simulink model "Automated_model_features"  (R2020b)
settings: Solver=VariableStepAuto  StartTime=0.0  StopTime=10.0  RelTol=1e-3
undefined symbols (not defined in the file): sigbuilder_block
libraries: simulink x123
(part 2 of 2)

== system Automated_model_features/MODULES/Tire Pressure Monitoring System/TP_Monitoring/indicateHigh1 ==
  Enable : EnablePort
  Constant : Constant  Value=0
  Out1 : Outport
  wires:
  Constant/1 -> Out1/1

== system Automated_model_features/MODULES/Tire Pressure Monitoring System/TP_Monitoring/indicateHigh2 ==
  Enable : EnablePort
  Constant : Constant  Value=0
  Out1 : Outport
  wires:
  Constant/1 -> Out1/1

== system Automated_model_features/MODULES/Tire Pressure Monitoring System/TP_Monitoring/indicateHigh3 ==
  Enable : EnablePort
  Constant : Constant  Value=0
  Out1 : Outport
  wires:
  Constant/1 -> Out1/1

== system Automated_model_features/MODULES/Tire Pressure Monitoring System/TP_Monitoring/indicateHigh4 ==
  Enable : EnablePort
  Constant : Constant  Value=0
  Out1 : Outport
  wires:
  Constant/1 -> Out1/1

== system Automated_model_features/MODULES/Tire Pressure Monitoring System/TP_Monitoring/indicateLow1 ==
  Enable : EnablePort
  Constant : Constant
  Out1 : Outport
  wires:
  Constant/1 -> Out1/1

== system Automated_model_features/MODULES/Tire Pressure Monitoring System/TP_Monitoring/indicateLow2 ==
  Enable : EnablePort
  Constant : Constant
  Out1 : Outport
  wires:
  Constant/1 -> Out1/1

== system Automated_model_features/MODULES/Tire Pressure Monitoring System/TP_Monitoring/indicateLow3 ==
  Enable : EnablePort
  Constant : Constant
  Out1 : Outport
  wires:
  Constant/1 -> Out1/1

== system Automated_model_features/MODULES/Tire Pressure Monitoring System/TP_Monitoring/indicateLow4 ==
  Enable : EnablePort
  Constant : Constant
  Out1 : Outport
  wires:
  Constant/1 -> Out1/1

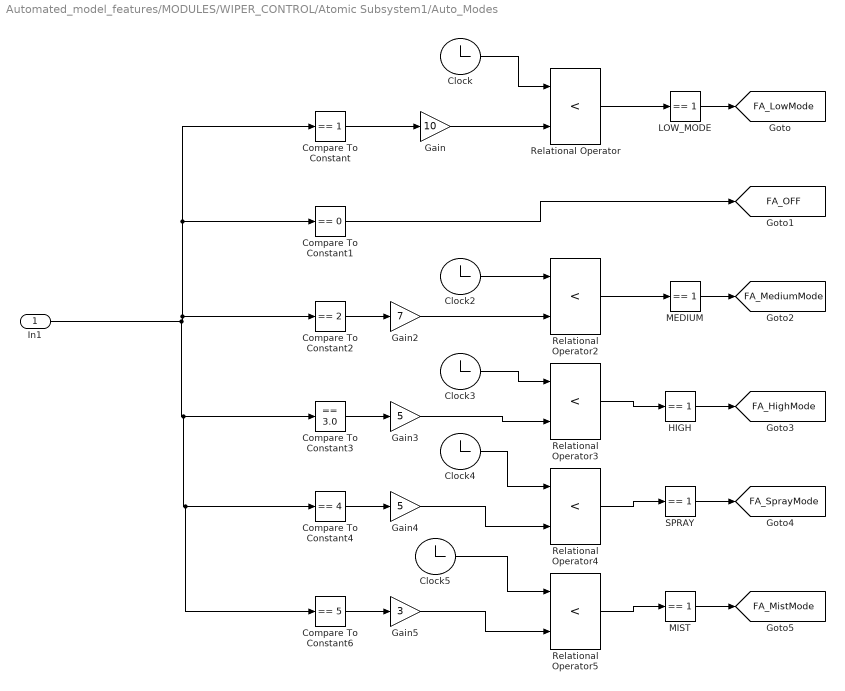
== system Automated_model_features/MODULES/WIPER_CONTROL/Atomic Subsystem1/Auto_Modes ==
  In1 : Inport
  Clock{,2..5} (5 alike) : Clock
      settings: Decimation=5
  Compare To Constant : simulink/Logic and Bit Operations/Compare To Constant  relop===  const=1  OutDataTypeStr=boolean
  Compare To Constant1 : simulink/Logic and Bit Operations/Compare To Constant  relop===  const=0  OutDataTypeStr=boolean
  Compare To Constant2 : simulink/Logic and Bit Operations/Compare To Constant  relop===  const=2  OutDataTypeStr=boolean
  Compare To Constant3 : simulink/Logic and Bit Operations/Compare To Constant  relop===  const=3.0  OutDataTypeStr=boolean
  Compare To Constant4 : simulink/Logic and Bit Operations/Compare To Constant  relop===  const=4  OutDataTypeStr=boolean
  Compare To Constant6 : simulink/Logic and Bit Operations/Compare To Constant  relop===  const=5  OutDataTypeStr=boolean
  Gain : Gain  Gain=10
  Gain2 : Gain  Gain=7
  Gain3 : Gain  Gain=5
  Gain4 : Gain  Gain=5
  Gain5 : Gain  Gain=3
  HIGH : simulink/Logic and Bit Operations/Compare To Constant  relop===  const=1  OutDataTypeStr=boolean
  LOW_MODE : simulink/Logic and Bit Operations/Compare To Constant  relop===  const=1  OutDataTypeStr=boolean
  MEDIUM : simulink/Logic and Bit Operations/Compare To Constant  relop===  const=1  OutDataTypeStr=boolean
  MIST : simulink/Logic and Bit Operations/Compare To Constant  relop===  const=1  OutDataTypeStr=boolean
  Relational Operator{,2..5} (5 alike) : RelationalOperator  Operator=<  OutDataTypeStr=boolean  RndMeth=Simplest
  SPRAY : simulink/Logic and Bit Operations/Compare To Constant  relop===  const=1  OutDataTypeStr=boolean
  tag scope: FA_HighMode=global, FA_LowMode=global, FA_MediumMode=global, FA_MistMode=global, FA_OFF=global, FA_SprayMode=global
  wires:
  In1/1 -> Compare To Constant6/1, Compare To Constant4/1, Compare To Constant3/1, Compare To Constant2/1, Compare To Constant/1, Compare To Constant1/1
  Clock/1 -> Relational Operator/1
  Relational Operator/1 -> LOW_MODE/1
  Gain/1 -> Relational Operator/2
  Compare To Constant/1 -> Gain/1
  Clock2/1 -> Relational Operator2/1
  Gain2/1 -> Relational Operator2/2
  Compare To Constant2/1 -> Gain2/1
  Clock3/1 -> Relational Operator3/1
  Gain3/1 -> Relational Operator3/2
  Compare To Constant3/1 -> Gain3/1
  Gain4/1 -> Relational Operator4/2
  Clock4/1 -> Relational Operator4/1
  Compare To Constant4/1 -> Gain4/1
  LOW_MODE/1 -> [FA_LowMode]
  MEDIUM/1 -> [FA_MediumMode]
  Relational Operator2/1 -> MEDIUM/1
  HIGH/1 -> [FA_HighMode]
  Relational Operator3/1 -> HIGH/1
  SPRAY/1 -> [FA_SprayMode]
  Relational Operator4/1 -> SPRAY/1
  Compare To Constant1/1 -> [FA_OFF]
  Relational Operator5/1 -> MIST/1
  Gain5/1 -> Relational Operator5/2
  Clock5/1 -> Relational Operator5/1
  MIST/1 -> [FA_MistMode]
  Compare To Constant6/1 -> Gain5/1

== system Automated_model_features/MODULES/WIPER_CONTROL/Atomic Subsystem1/Manual_mode ==
  In1 : Inport
  Bw30_60 : Logic  IconShape=distinctive  AllPortsSameDT=off  OutDataTypeStr=boolean
  Bw60_100 : Logic  IconShape=distinctive  AllPortsSameDT=off  OutDataTypeStr=boolean
  Compare To Constant1 : simulink/Logic and Bit Operations/Compare To Constant  relop=>  const=30  OutDataTypeStr=boolean
  Compare To Constant2 : simulink/Logic and Bit Operations/Compare To Constant  relop=<=  const=60  OutDataTypeStr=boolean
  Compare To Constant3 : simulink/Logic and Bit Operations/Compare To Constant  relop=>  const=60  OutDataTypeStr=boolean
  Compare To Constant4 : simulink/Logic and Bit Operations/Compare To Constant  relop=<=  const=100  OutDataTypeStr=boolean
  Display : Display
  LessThan30 : simulink/Logic and Bit Operations/Compare To Constant  relop=<=  const=30  OutDataTypeStr=boolean
  Slider : SliderBlock
  String Constant : StringConstant  String="\"Undefined!\""
  Switch : Switch  Criteria=u2 > Threshold  Threshold=5
  tag scope: FM_Bw30_60=global, FM_Bw60_100=global, FM_lessthan30=global
  wires:
  Compare To Constant1/1 -> Bw30_60/1
  Bw30_60/1 -> [FM_Bw30_60]
  [FC_ManualInput] -> Compare To Constant4/1, Compare To Constant3/1, Compare To Constant2/1, Compare To Constant1/1, LessThan30/1, Switch/1
  Compare To Constant4/1 -> Bw60_100/2
  LessThan30/1 -> [FM_lessthan30]
  Switch/1 -> Display/1
  Compare To Constant3/1 -> Bw60_100/1
  Bw60_100/1 -> [FM_Bw60_100]
  Compare To Constant2/1 -> Bw30_60/2
  In1/1 -> Switch/2
  String Constant/1 -> Switch/3

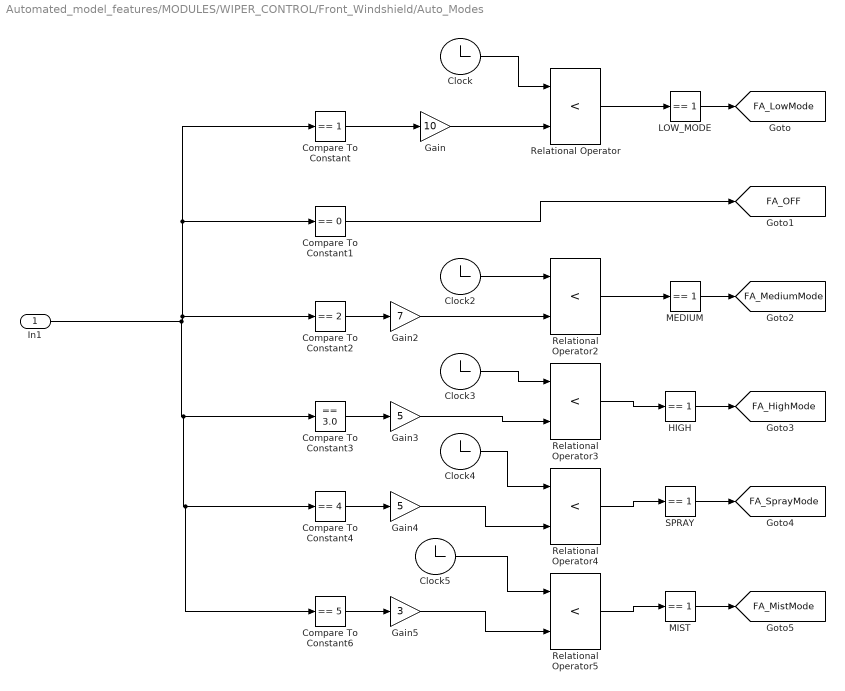
== system Automated_model_features/MODULES/WIPER_CONTROL/Front_Windshield/Auto_Modes ==
  In1 : Inport
  Clock{,2..5} (5 alike) : Clock
      settings: Decimation=5
  Compare To Constant : simulink/Logic and Bit Operations/Compare To Constant  relop===  const=1  OutDataTypeStr=boolean
  Compare To Constant1 : simulink/Logic and Bit Operations/Compare To Constant  relop===  const=0  OutDataTypeStr=boolean
  Compare To Constant2 : simulink/Logic and Bit Operations/Compare To Constant  relop===  const=2  OutDataTypeStr=boolean
  Compare To Constant3 : simulink/Logic and Bit Operations/Compare To Constant  relop===  const=3.0  OutDataTypeStr=boolean
  Compare To Constant4 : simulink/Logic and Bit Operations/Compare To Constant  relop===  const=4  OutDataTypeStr=boolean
  Compare To Constant6 : simulink/Logic and Bit Operations/Compare To Constant  relop===  const=5  OutDataTypeStr=boolean
  Gain : Gain  Gain=10
  Gain2 : Gain  Gain=7
  Gain3 : Gain  Gain=5
  Gain4 : Gain  Gain=5
  Gain5 : Gain  Gain=3
  HIGH : simulink/Logic and Bit Operations/Compare To Constant  relop===  const=1  OutDataTypeStr=boolean
  LOW_MODE : simulink/Logic and Bit Operations/Compare To Constant  relop===  const=1  OutDataTypeStr=boolean
  MEDIUM : simulink/Logic and Bit Operations/Compare To Constant  relop===  const=1  OutDataTypeStr=boolean
  MIST : simulink/Logic and Bit Operations/Compare To Constant  relop===  const=1  OutDataTypeStr=boolean
  Relational Operator{,2..5} (5 alike) : RelationalOperator  Operator=<  OutDataTypeStr=boolean  RndMeth=Simplest
  SPRAY : simulink/Logic and Bit Operations/Compare To Constant  relop===  const=1  OutDataTypeStr=boolean
  tag scope: FA_HighMode=global, FA_LowMode=global, FA_MediumMode=global, FA_MistMode=global, FA_OFF=global, FA_SprayMode=global
  wires:
  In1/1 -> Compare To Constant6/1, Compare To Constant4/1, Compare To Constant3/1, Compare To Constant2/1, Compare To Constant/1, Compare To Constant1/1
  Clock/1 -> Relational Operator/1
  Relational Operator/1 -> LOW_MODE/1
  Gain/1 -> Relational Operator/2
  Compare To Constant/1 -> Gain/1
  Clock2/1 -> Relational Operator2/1
  Gain2/1 -> Relational Operator2/2
  Compare To Constant2/1 -> Gain2/1
  Clock3/1 -> Relational Operator3/1
  Gain3/1 -> Relational Operator3/2
  Compare To Constant3/1 -> Gain3/1
  Gain4/1 -> Relational Operator4/2
  Clock4/1 -> Relational Operator4/1
  Compare To Constant4/1 -> Gain4/1
  LOW_MODE/1 -> [FA_LowMode]
  MEDIUM/1 -> [FA_MediumMode]
  Relational Operator2/1 -> MEDIUM/1
  HIGH/1 -> [FA_HighMode]
  Relational Operator3/1 -> HIGH/1
  SPRAY/1 -> [FA_SprayMode]
  Relational Operator4/1 -> SPRAY/1
  Compare To Constant1/1 -> [FA_OFF]
  Relational Operator5/1 -> MIST/1
  Gain5/1 -> Relational Operator5/2
  Clock5/1 -> Relational Operator5/1
  MIST/1 -> [FA_MistMode]
  Compare To Constant6/1 -> Gain5/1

== system Automated_model_features/MODULES/WIPER_CONTROL/Front_Windshield/Manual_mode ==
  In1 : Inport
  Bw30_60 : Logic  IconShape=distinctive  AllPortsSameDT=off  OutDataTypeStr=boolean
  Bw60_100 : Logic  IconShape=distinctive  AllPortsSameDT=off  OutDataTypeStr=boolean
  Compare To Constant1 : simulink/Logic and Bit Operations/Compare To Constant  relop=>  const=30  OutDataTypeStr=boolean
  Compare To Constant2 : simulink/Logic and Bit Operations/Compare To Constant  relop=<=  const=60  OutDataTypeStr=boolean
  Compare To Constant3 : simulink/Logic and Bit Operations/Compare To Constant  relop=>  const=60  OutDataTypeStr=boolean
  Compare To Constant4 : simulink/Logic and Bit Operations/Compare To Constant  relop=<=  const=100  OutDataTypeStr=boolean
  Display : Display
  LessThan30 : simulink/Logic and Bit Operations/Compare To Constant  relop=<=  const=30  OutDataTypeStr=boolean
  Slider : SliderBlock
  String Constant : StringConstant  String="\"Undefined!\""
  Switch : Switch  Criteria=u2 > Threshold  Threshold=5
  tag scope: FM_Bw30_60=global, FM_Bw60_100=global, FM_lessthan30=global
  wires:
  Compare To Constant1/1 -> Bw30_60/1
  Bw30_60/1 -> [FM_Bw30_60]
  [FC_ManualInput] -> Compare To Constant4/1, Compare To Constant3/1, Compare To Constant2/1, Compare To Constant1/1, LessThan30/1, Switch/1
  Compare To Constant4/1 -> Bw60_100/2
  LessThan30/1 -> [FM_lessthan30]
  Switch/1 -> Display/1
  Compare To Constant3/1 -> Bw60_100/1
  Bw60_100/1 -> [FM_Bw60_100]
  Compare To Constant2/1 -> Bw30_60/2
  In1/1 -> Switch/2
  String Constant/1 -> Switch/3

== system Automated_model_features/MODULES/WIPER_CONTROL/Wiper_Control/Atomic Subsystem ==
  Inport : Inport
  Clock : Clock
      settings: Decimation=5
  Compare To Constant : simulink/Logic and Bit Operations/Compare To Constant  relop===  const=1  OutDataTypeStr=boolean
  Compare To Constant5 : simulink/Logic and Bit Operations/Compare To Constant  relop===  const=1  OutDataTypeStr=boolean
  Gain : Gain  Gain=10
  Relational Operator : RelationalOperator  Operator=<  OutDataTypeStr=boolean  RndMeth=Simplest
  tag scope: BW_Display=global
  wires:
  Compare To Constant5/1 -> [BW_Display]
  Inport/1 -> Compare To Constant/1
  Gain/1 -> Relational Operator/2
  Clock/1 -> Relational Operator/1
  Relational Operator/1 -> Compare To Constant5/1
  Compare To Constant/1 -> Gain/1

== system Automated_model_features/MODULES/WIPER_CONTROL/Wiper_Control/Atomic Subsystem1 ==
  Inport : Inport
  Auto_Modes : Subsystem
  Display : Display
  Manual_mode : Subsystem
  wires:
  [FW_Modes] -> Manual_mode/1(In1), Auto_Modes/1(In1)
  Inport/1 -> Display/1

== system Automated_model_features/MODULES/WIPER_CONTROL/Wiper_Control/Back_Windshield ==
  Lamp : LampBlock

== system Automated_model_features/MODULES/WIPER_CONTROL/Wiper_Control/Front_Windshield ==
  Enable : EnablePort
  Auto_Modes : Subsystem
  Manual_mode : Subsystem
  Rotary Switch : RotarySwitchBlock  Commented=on
      settings: Values={{'Off', 'Low', 'Medium', 'High', 'Spray', 'Manual', 'MistMode'}, [0 1 2 3 4 5 6]}
  wires:
  [FW_Modes] -> Manual_mode/1(In1), Auto_Modes/1(In1)

== system Automated_model_features/MODULES/sunroof/Subsystem/Enabled Subsystem ==
  In1 : Inport
  Enable : EnablePort
  Outport : Outport
  wires:
  In1/1 -> Outport/1

== system Automated_model_features/MODULES/sunroof/Subsystem1/Enabled Subsystem1 ==
  In1 : Inport
  Enable : EnablePort
  Outport : Outport
  wires:
  In1/1 -> Outport/1

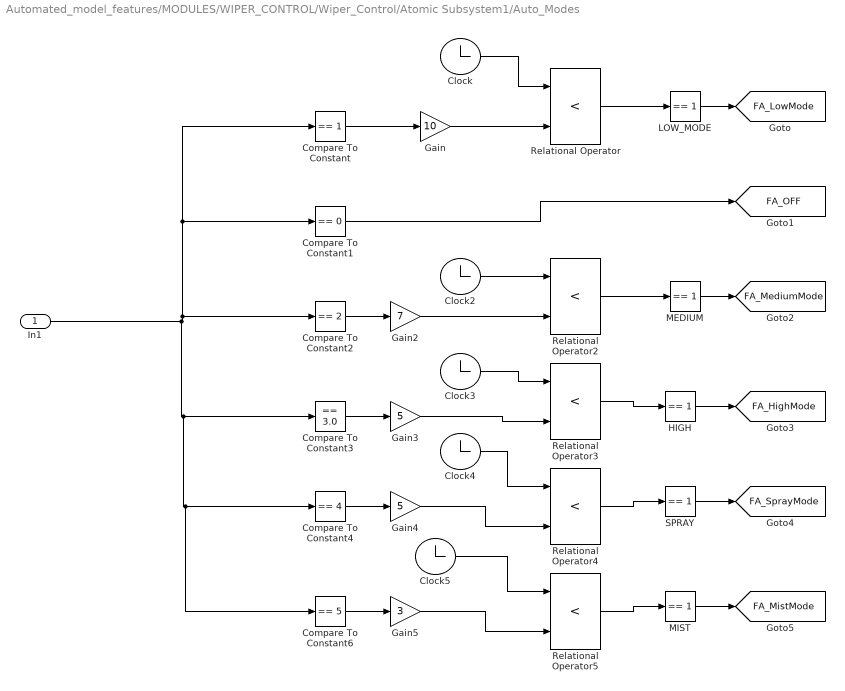
== system Automated_model_features/MODULES/WIPER_CONTROL/Wiper_Control/Atomic Subsystem1/Auto_Modes ==
  In1 : Inport
  Clock{,2..5} (5 alike) : Clock
      settings: Decimation=5
  Compare To Constant : simulink/Logic and Bit Operations/Compare To Constant  relop===  const=1  OutDataTypeStr=boolean
  Compare To Constant1 : simulink/Logic and Bit Operations/Compare To Constant  relop===  const=0  OutDataTypeStr=boolean
  Compare To Constant2 : simulink/Logic and Bit Operations/Compare To Constant  relop===  const=2  OutDataTypeStr=boolean
  Compare To Constant3 : simulink/Logic and Bit Operations/Compare To Constant  relop===  const=3.0  OutDataTypeStr=boolean
  Compare To Constant4 : simulink/Logic and Bit Operations/Compare To Constant  relop===  const=4  OutDataTypeStr=boolean
  Compare To Constant6 : simulink/Logic and Bit Operations/Compare To Constant  relop===  const=5  OutDataTypeStr=boolean
  Gain : Gain  Gain=10
  Gain2 : Gain  Gain=7
  Gain3 : Gain  Gain=5
  Gain4 : Gain  Gain=5
  Gain5 : Gain  Gain=3
  HIGH : simulink/Logic and Bit Operations/Compare To Constant  relop===  const=1  OutDataTypeStr=boolean
  LOW_MODE : simulink/Logic and Bit Operations/Compare To Constant  relop===  const=1  OutDataTypeStr=boolean
  MEDIUM : simulink/Logic and Bit Operations/Compare To Constant  relop===  const=1  OutDataTypeStr=boolean
  MIST : simulink/Logic and Bit Operations/Compare To Constant  relop===  const=1  OutDataTypeStr=boolean
  Relational Operator{,2..5} (5 alike) : RelationalOperator  Operator=<  OutDataTypeStr=boolean  RndMeth=Simplest
  SPRAY : simulink/Logic and Bit Operations/Compare To Constant  relop===  const=1  OutDataTypeStr=boolean
  tag scope: FA_HighMode=global, FA_LowMode=global, FA_MediumMode=global, FA_MistMode=global, FA_OFF=global, FA_SprayMode=global
  wires:
  In1/1 -> Compare To Constant6/1, Compare To Constant4/1, Compare To Constant3/1, Compare To Constant2/1, Compare To Constant/1, Compare To Constant1/1
  Clock/1 -> Relational Operator/1
  Relational Operator/1 -> LOW_MODE/1
  Gain/1 -> Relational Operator/2
  Compare To Constant/1 -> Gain/1
  Clock2/1 -> Relational Operator2/1
  Gain2/1 -> Relational Operator2/2
  Compare To Constant2/1 -> Gain2/1
  Clock3/1 -> Relational Operator3/1
  Gain3/1 -> Relational Operator3/2
  Compare To Constant3/1 -> Gain3/1
  Gain4/1 -> Relational Operator4/2
  Clock4/1 -> Relational Operator4/1
  Compare To Constant4/1 -> Gain4/1
  LOW_MODE/1 -> [FA_LowMode]
  MEDIUM/1 -> [FA_MediumMode]
  Relational Operator2/1 -> MEDIUM/1
  HIGH/1 -> [FA_HighMode]
  Relational Operator3/1 -> HIGH/1
  SPRAY/1 -> [FA_SprayMode]
  Relational Operator4/1 -> SPRAY/1
  Compare To Constant1/1 -> [FA_OFF]
  Relational Operator5/1 -> MIST/1
  Gain5/1 -> Relational Operator5/2
  Clock5/1 -> Relational Operator5/1
  MIST/1 -> [FA_MistMode]
  Compare To Constant6/1 -> Gain5/1

== system Automated_model_features/MODULES/WIPER_CONTROL/Wiper_Control/Atomic Subsystem1/Manual_mode ==
  In1 : Inport
  Bw30_60 : Logic  IconShape=distinctive  AllPortsSameDT=off  OutDataTypeStr=boolean
  Bw60_100 : Logic  IconShape=distinctive  AllPortsSameDT=off  OutDataTypeStr=boolean
  Compare To Constant1 : simulink/Logic and Bit Operations/Compare To Constant  relop=>  const=30  OutDataTypeStr=boolean
  Compare To Constant2 : simulink/Logic and Bit Operations/Compare To Constant  relop=<=  const=60  OutDataTypeStr=boolean
  Compare To Constant3 : simulink/Logic and Bit Operations/Compare To Constant  relop=>  const=60  OutDataTypeStr=boolean
  Compare To Constant4 : simulink/Logic and Bit Operations/Compare To Constant  relop=<=  const=100  OutDataTypeStr=boolean
  Display : Display
  LessThan30 : simulink/Logic and Bit Operations/Compare To Constant  relop=<=  const=30  OutDataTypeStr=boolean
  Slider : SliderBlock
  String Constant : StringConstant  String="\"Undefined!\""
  Switch : Switch  Criteria=u2 > Threshold  Threshold=5
  tag scope: FM_Bw30_60=global, FM_Bw60_100=global, FM_lessthan30=global
  wires:
  Compare To Constant1/1 -> Bw30_60/1
  Bw30_60/1 -> [FM_Bw30_60]
  [FC_ManualInput] -> Compare To Constant4/1, Compare To Constant3/1, Compare To Constant2/1, Compare To Constant1/1, LessThan30/1, Switch/1
  Compare To Constant4/1 -> Bw60_100/2
  LessThan30/1 -> [FM_lessthan30]
  Switch/1 -> Display/1
  Compare To Constant3/1 -> Bw60_100/1
  Bw60_100/1 -> [FM_Bw60_100]
  Compare To Constant2/1 -> Bw30_60/2
  In1/1 -> Switch/2
  String Constant/1 -> Switch/3

== system Automated_model_features/MODULES/WIPER_CONTROL/Wiper_Control/Front_Windshield/Auto_Modes ==
  In1 : Inport
  Clock{,2..5} (5 alike) : Clock
      settings: Decimation=5
  Compare To Constant : simulink/Logic and Bit Operations/Compare To Constant  relop===  const=1  OutDataTypeStr=boolean
  Compare To Constant1 : simulink/Logic and Bit Operations/Compare To Constant  relop===  const=0  OutDataTypeStr=boolean
  Compare To Constant2 : simulink/Logic and Bit Operations/Compare To Constant  relop===  const=2  OutDataTypeStr=boolean
  Compare To Constant3 : simulink/Logic and Bit Operations/Compare To Constant  relop===  const=3.0  OutDataTypeStr=boolean
  Compare To Constant4 : simulink/Logic and Bit Operations/Compare To Constant  relop===  const=4  OutDataTypeStr=boolean
  Compare To Constant6 : simulink/Logic and Bit Operations/Compare To Constant  relop===  const=5  OutDataTypeStr=boolean
  Gain : Gain  Gain=10
  Gain2 : Gain  Gain=7
  Gain3 : Gain  Gain=5
  Gain4 : Gain  Gain=5
  Gain5 : Gain  Gain=3
  HIGH : simulink/Logic and Bit Operations/Compare To Constant  relop===  const=1  OutDataTypeStr=boolean
  LOW_MODE : simulink/Logic and Bit Operations/Compare To Constant  relop===  const=1  OutDataTypeStr=boolean
  MEDIUM : simulink/Logic and Bit Operations/Compare To Constant  relop===  const=1  OutDataTypeStr=boolean
  MIST : simulink/Logic and Bit Operations/Compare To Constant  relop===  const=1  OutDataTypeStr=boolean
  Relational Operator{,2..5} (5 alike) : RelationalOperator  Operator=<  OutDataTypeStr=boolean  RndMeth=Simplest
  SPRAY : simulink/Logic and Bit Operations/Compare To Constant  relop===  const=1  OutDataTypeStr=boolean
  tag scope: FA_HighMode=global, FA_LowMode=global, FA_MediumMode=global, FA_MistMode=global, FA_OFF=global, FA_SprayMode=global
  wires:
  In1/1 -> Compare To Constant6/1, Compare To Constant4/1, Compare To Constant3/1, Compare To Constant2/1, Compare To Constant/1, Compare To Constant1/1
  Clock/1 -> Relational Operator/1
  Relational Operator/1 -> LOW_MODE/1
  Gain/1 -> Relational Operator/2
  Compare To Constant/1 -> Gain/1
  Clock2/1 -> Relational Operator2/1
  Gain2/1 -> Relational Operator2/2
  Compare To Constant2/1 -> Gain2/1
  Clock3/1 -> Relational Operator3/1
  Gain3/1 -> Relational Operator3/2
  Compare To Constant3/1 -> Gain3/1
  Gain4/1 -> Relational Operator4/2
  Clock4/1 -> Relational Operator4/1
  Compare To Constant4/1 -> Gain4/1
  LOW_MODE/1 -> [FA_LowMode]
  MEDIUM/1 -> [FA_MediumMode]
  Relational Operator2/1 -> MEDIUM/1
  HIGH/1 -> [FA_HighMode]
  Relational Operator3/1 -> HIGH/1
  SPRAY/1 -> [FA_SprayMode]
  Relational Operator4/1 -> SPRAY/1
  Compare To Constant1/1 -> [FA_OFF]
  Relational Operator5/1 -> MIST/1
  Gain5/1 -> Relational Operator5/2
  Clock5/1 -> Relational Operator5/1
  MIST/1 -> [FA_MistMode]
  Compare To Constant6/1 -> Gain5/1

== system Automated_model_features/MODULES/WIPER_CONTROL/Wiper_Control/Front_Windshield/Manual_mode ==
  In1 : Inport
  Bw30_60 : Logic  IconShape=distinctive  AllPortsSameDT=off  OutDataTypeStr=boolean
  Bw60_100 : Logic  IconShape=distinctive  AllPortsSameDT=off  OutDataTypeStr=boolean
  Compare To Constant1 : simulink/Logic and Bit Operations/Compare To Constant  relop=>  const=30  OutDataTypeStr=boolean
  Compare To Constant2 : simulink/Logic and Bit Operations/Compare To Constant  relop=<=  const=60  OutDataTypeStr=boolean
  Compare To Constant3 : simulink/Logic and Bit Operations/Compare To Constant  relop=>  const=60  OutDataTypeStr=boolean
  Compare To Constant4 : simulink/Logic and Bit Operations/Compare To Constant  relop=<=  const=100  OutDataTypeStr=boolean
  Display : Display
  LessThan30 : simulink/Logic and Bit Operations/Compare To Constant  relop=<=  const=30  OutDataTypeStr=boolean
  Slider : SliderBlock
  String Constant : StringConstant  String="\"Undefined!\""
  Switch : Switch  Criteria=u2 > Threshold  Threshold=5
  tag scope: FM_Bw30_60=global, FM_Bw60_100=global, FM_lessthan30=global
  wires:
  Compare To Constant1/1 -> Bw30_60/1
  Bw30_60/1 -> [FM_Bw30_60]
  [FC_ManualInput] -> Compare To Constant4/1, Compare To Constant3/1, Compare To Constant2/1, Compare To Constant1/1, LessThan30/1, Switch/1
  Compare To Constant4/1 -> Bw60_100/2
  LessThan30/1 -> [FM_lessthan30]
  Switch/1 -> Display/1
  Compare To Constant3/1 -> Bw60_100/1
  Bw60_100/1 -> [FM_Bw60_100]
  Compare To Constant2/1 -> Bw30_60/2
  In1/1 -> Switch/2
  String Constant/1 -> Switch/3

== stateflow chart Automated_model_features/MODULES/ALARM_SYSTEM/Pre_Alarm ==
  state RKE1
    entry:
  state DELAY_3
    entry:
    data1 = 1;
  state DELAY_2
    entry:
    counter=0;
    counter = counter +1;
    data1 = 0;
  (default) -> RKE1
  RKE1 -> DELAY_3 [order 2] : [data==1]
  RKE1 -> DELAY_2 [order 1] : [data==0]
  DELAY_2 -> DELAY_2 : [counter~=10]
  data: data input; data1 output; counter local

== stateflow chart Automated_model_features/MODULES/sunroof/enabling system/Chart ==
  state stage1
    entry:
    enableO=0;
    enableC=0;
  state stage3
    entry:
    enableO=1;
    enableC=0;
  state stage2
    entry:
    enableO=0;
    enableC=1;
  (default) -> stage1
  stage1 -> stage3 [order 3] : [openButton ==1 && closeButton==0]
  stage1 -> stage2 [order 1] : [openButton ==0 && closeButton==1]
  stage2 -> stage1 : [(openButton ==1 && closeButton==1) || (openButton ==0 && closeButton==0)]
  stage3 -> stage1 : [(openButton ==1 && closeButton==1) || (openButton ==0 && closeButton==0)]
  stage1 -> stage1 [order 2] : [(openButton ==1 && closeButton==1) || (openButton ==0 && closeButton==0)]
  data: closeButton input; openButton input; enableC output; enableO output

== matlab function Automated_model_features/MODULES/AIRBAGSYSTEM/ActivateAirBagSensor ==
  data: SuddenDeceleration input; AirBagSensor output
function AirBagSensor  = fcn(SuddenDeceleration)
if SuddenDeceleration == 1
         %Front airbag active
   AirBagSensor = 1;
else 
   AirBagSensor = 0;   
end

== matlab function Automated_model_features/MODULES/AIRBAGSYSTEM/FrontAirBagActivation/WeightSensor ==
  data: driver input; DRIVER output; l_front input; L_FRONT output; l_rear input; r_rear input; L_REAR output; R_REAR output
function [DRIVER,L_FRONT,L_REAR,R_REAR] = fcn(driver, l_front,l_rear,r_rear)
    if (driver==0 && l_front==0 && l_rear==0 && r_rear==1)      %0001
        DRIVER=0;
        L_FRONT=0;
        L_REAR=0;
        R_REAR=1;
    
    elseif (driver==0 && l_front==0 && l_rear==1 && r_rear==0)
        DRIVER=0;
        L_FRONT=0;
        L_REAR=1;
        R_REAR=0;
    
    elseif (driver==0 && l_front==0 && l_rear==1 && r_rear==1)
        DRIVER=0;
        L_FRONT=0;
        L_REAR=1;
        R_REAR=1;

    elseif (driver==0 && l_front==1 && l_rear==0 && r_rear==0)
        DRIVER=0;
        L_FRONT=1;
        L_REAR=0;
        R_REAR=0;
    
    elseif (driver==0 && l_front==1 && l_rear==0 && r_rear==1)
        DRIVER=0;
        L_FRONT=1;
        L_REAR=0;
        R_REAR=1;
    
    elseif (driver==0 && l_front==1 && l_rear==1 && r_rear==0)
        DRIVER=0;
        L_FRONT=1;
        L_REAR=1;
        R_REAR=0;
    
    elseif (driver==0 && l_front==1 && l_rear==1 && r_rear==1)
        DRIVER=0;
        L_FRONT=1;
        L_REAR=1;
        R_REAR=1;
    
    elseif (driver==1 && l_front==0 && l_rear==0 && r_rear==0)
        DRIVER=1;
        L_FRONT=0;
        L_REAR=0;
        R_REAR=0;
    
    elseif (driver==1 && l_front==0 && l_rear==0 && r_rear==1)
        DRIVER=1;
        L_FRONT=0;
        L_REAR=0;
        R_REAR=1;
    
    elseif (driver==1 && l_front==0 && l_rear==1 && r_rear==0)
        DRIVER=1;
        L_FRONT=0;
        L_REAR=1;
        R_REAR=0;
    
    elseif (driver==1 && l_front==0 && l_rear==1 && r_rear==1)
        DRIVER=1;
        L_FRONT=0;
        L_REAR=1;
        R_REAR=1;
    
    elseif (driver==1 && l_front==1 && l_rear==0 && r_rear==0)
        DRIVER=1;
        L_FRONT=1;
        L_REAR=0;
        R_REAR=0;
    
    elseif (driver==1 && l_front==1 && l_rear==0 && r_rear==1)
        DRIVER=1;
        L_FRONT=1;
        L_REAR=0;
        R_REAR=1;
    
    elseif (driver==1 && l_front==1 && l_rear==1 && r_rear==0)
        DRIVER=1;
        L_FRONT=1;
        L_REAR=1;
        R_REAR=0;
    
    elseif (driver==1 && l_front==1 && l_rear==1 && r_rear==1)
        DRIVER=1;
        L_FRONT=1;
        L_REAR=1;
        R_REAR=1;
    
    else
        DRIVER=0;
        L_FRONT=0;
        L_REAR=0;
        R_REAR=0;
    end

== matlab function Automated_model_features/MODULES/AIRBAGSYSTEM/SideAirBagActivation1/WeightSensor ==
  data: driver input; DRIVER output; l_front input; L_FRONT output; l_rear input; r_rear input; L_REAR output; R_REAR output
function [DRIVER,L_FRONT,L_REAR,R_REAR] = fcn(driver, l_front,l_rear,r_rear)
    if (driver==0 && l_front==0 && l_rear==0 && r_rear==1)      %0001
        DRIVER=0;
        L_FRONT=0;
        L_REAR=0;
        R_REAR=1;
    
    elseif (driver==0 && l_front==0 && l_rear==1 && r_rear==0)
        DRIVER=0;
        L_FRONT=0;
        L_REAR=1;
        R_REAR=0;
    
    elseif (driver==0 && l_front==0 && l_rear==1 && r_rear==1)
        DRIVER=0;
        L_FRONT=0;
        L_REAR=1;
        R_REAR=1;

    elseif (driver==0 && l_front==1 && l_rear==0 && r_rear==0)
        DRIVER=0;
        L_FRONT=1;
        L_REAR=0;
        R_REAR=0;
    
    elseif (driver==0 && l_front==1 && l_rear==0 && r_rear==1)
        DRIVER=0;
        L_FRONT=1;
        L_REAR=0;
        R_REAR=1;
    
    elseif (driver==0 && l_front==1 && l_rear==1 && r_rear==0)
        DRIVER=0;
        L_FRONT=1;
        L_REAR=1;
        R_REAR=0;
    
    elseif (driver==0 && l_front==1 && l_rear==1 && r_rear==1)
        DRIVER=0;
        L_FRONT=1;
        L_REAR=1;
        R_REAR=1;
    
    elseif (driver==1 && l_front==0 && l_rear==0 && r_rear==0)
        DRIVER=1;
        L_FRONT=0;
        L_REAR=0;
        R_REAR=0;
    
    elseif (driver==1 && l_front==0 && l_rear==0 && r_rear==1)
        DRIVER=1;
        L_FRONT=0;
        L_REAR=0;
        R_REAR=1;
    
    elseif (driver==1 && l_front==0 && l_rear==1 && r_rear==0)
        DRIVER=1;
        L_FRONT=0;
        L_REAR=1;
        R_REAR=0;
    
    elseif (driver==1 && l_front==0 && l_rear==1 && r_rear==1)
        DRIVER=1;
        L_FRONT=0;
        L_REAR=1;
        R_REAR=1;
    
    elseif (driver==1 && l_front==1 && l_rear==0 && r_rear==0)
        DRIVER=1;
        L_FRONT=1;
        L_REAR=0;
        R_REAR=0;
    
    elseif (driver==1 && l_front==1 && l_rear==0 && r_rear==1)
        DRIVER=1;
        L_FRONT=1;
        L_REAR=0;
        R_REAR=1;
    
    elseif (driver==1 && l_front==1 && l_rear==1 && r_rear==0)
        DRIVER=1;
        L_FRONT=1;
        L_REAR=1;
        R_REAR=0;
    
    elseif (driver==1 && l_front==1 && l_rear==1 && r_rear==1)
        DRIVER=1;
        L_FRONT=1;
        L_REAR=1;
        R_REAR=1;
    
    else
        DRIVER=0;
        L_FRONT=0;
        L_REAR=0;
        R_REAR=0;
    end

== stateflow chart Automated_model_features/MODULES/ALARM_SYSTEM/ARMED ==
  state data
  state DELAY_1
    entry:
    data1 = 1;
  state DELAY
    entry:
    count=0;
    count = count + 1;
    data1 = 1;
  data -> DELAY_1 [order 2] : [data==1]
  (default) -> data
  data -> DELAY [order 1] : [data==0]
  DELAY -> DELAY : [count~=30]
  data: data input; data1 output; count local

== stateflow chart Automated_model_features/MODULES/ALARM_SYSTEM/Main_Alarm/ARMED ==
  state data
  state DELAY_1
    entry:
    data1 = 1;
  state DELAY
    entry:
    count=0;
    count = count + 1;
    data1 = 1;
  data -> DELAY_1 [order 2] : [data==1]
  (default) -> data
  data -> DELAY [order 1] : [data==0]
  DELAY -> DELAY : [count~=30]
  data: data input; data1 output; count local

== stateflow chart Automated_model_features/MODULES/ALARM_SYSTEM/Main_Alarm/Pre_Alarm ==
  state RKE1
    entry:
  state DELAY_3
    entry:
    data1 = 1;
  state DELAY_2
    entry:
    counter=0;
    counter = counter +1;
    data1 = 0;
  (default) -> RKE1
  RKE1 -> DELAY_3 [order 2] : [data==1]
  RKE1 -> DELAY_2 [order 1] : [data==0]
  DELAY_2 -> DELAY_2 : [counter~=10]
  data: data input; data1 output; counter local
